simulink library "PUMATRC_lib"  (Simulink 6.0)
settings: Solver=ode45  SolverMode=SingleTasking  StartTime=0.0  StopTime=10.0  RelTol=1e-3
settings Model: LastModifiedBy=martin
settings OptimizationCC: BooleanDataType=off
settings DebuggingCC: SolverPrmCheckMsg=none
settings HardwareCC: TargetUnknown=on

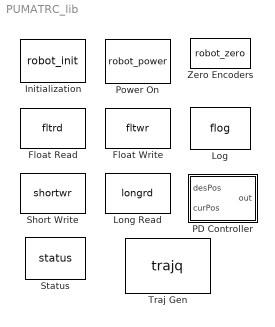
== system PUMATRC_lib ==
  Float Read : S-Function  Priority=10  FunctionName=fltrd  Parameters=option,channel,sampleTime  mask{option=TORQUE, channel=0, sampleTime=0}
      mask prompts: sampleTime "Sample Time"
      mask help: Reads a float value from OPTION offset and channel of Servo-To-Go board.
      mask StyleString: popup(TORQUE|TORQUE6|VOLTAGE|POSITION|POSITION6|STATUS|POT|POT6|INDEX|INDEX6|POWER|CALIB),edit,edit
      mask Display: port_label ('output',1,'val')
  Float Write : S-Function  Priority=10  FunctionName=fltwr  Parameters=option,channel,sampleTime  mask{option=TORQUE, channel=0, sampleTime=0}
      mask prompts: sampleTime "Sample Time"
      mask help: Writes a float value to OPTION offset and channel of Servo-To-Go board.
      mask StyleString: popup(TORQUE|TORQUE6|VOLTAGE|POSITION|POSITION6|STATUS|POT|POT6|INDEX|INDEX6|POWER|CALIB),edit,edit
      mask Display:
      | port_label('input',1,'val')
      | disp('')
  Initialization : S-Function  Priority=1  FunctionName=robot_init  Parameters=boardAddr  mask{boardAddr=0}
      mask prompts: boardAddr "Board Address(in decimal)"
      mask help: Initializes a Servo-To-Go board. Enter board address in decimal.
      mask Display: disp('Board\nInitialization')
  Log : S-Function  Priority=10  FunctionName=flog  Parameters=fileName,sampleTime  mask{fileName=0, sampleTime=0}
      mask prompts: fileName "Log Filename"; sampleTime "Sample Time"
      mask help: Values from the input are written to the filename at the specified period. The filename should be relative to the directory where model/code resides.
      mask Display:
      | port_label('input',1,'to File')
      | disp('')
  Long Read : S-Function  Priority=10  FunctionName=longrd  Parameters=option,channel,sampleTime  mask{option=TORQUE, channel=0, sampleTime=0}
      mask prompts: sampleTime "Sample Time"
      mask help: Writes a long value to OPTION offset and channel of Servo-To-Go board.
      mask StyleString: popup(TORQUE|TORQUE6|VOLTAGE|POSITION|POSITION6|STATUS|POT|POT6|INDEX|INDEX6|POWER|CALIB),edit,edit
      mask Display:
      | port_label('output',1,'val')
      | disp('')
  PD Controller : Subsystem  Priority=10  mask{Kp=0, Kd=0, T=0}
      mask prompts: T "Sample Time"
      mask help: Proportional-Derivative controller. Torque = Kp*(desPos- pos) - Kv*(time averaged velocity)
  Power On : S-Function  Priority=2  FunctionName=robot_power
      mask Display: disp('Power On')
  Short Write : S-Function  Priority=10  FunctionName=shortwr  Parameters=option,channel,sampleTime  mask{option=TORQUE, channel=0, sampleTime=0}
      mask prompts: sampleTime "Sample Time"
      mask help: Reads a short value from OPTION offset and channel of Servo-To-Go board.
      mask StyleString: popup(TORQUE|TORQUE6|VOLTAGE|POSITION|POSITION6|STATUS|POT|POT6|INDEX|INDEX6|POWER|CALIB),edit,edit
      mask Display:
      | port_label('input',1,'val')
      | disp('')
  Status : S-Function  FunctionName=status  Parameters=option,channel,sampleTime,  mask{option=TORQUE, channel=0, sampleTime=0}
      mask prompts: sampleTime "Sample Time"
      mask StyleString: popup(TORQUE|TORQUE6|VOLTAGE|POSITION|POSITION6|STATUS|POT|POT6|INDEX|INDEX6|POWER|CALIB|HAND|INDEX_BIT|ALL_INDEX_BITS|CLR_INDEX_BIT|CLR_INDEX_BITS|CLR_ADC_BIT ),edit,edit
      mask Display: port_label('output',1,'val')
  Traj Gen : S-Function  Priority=10  FunctionName=trajq  Parameters=sampleTime,jtMin,jtMax,calibFile,jtIncr  mask{sampleTime=0, jtMin=0, jtMax=0, calibFile=0, jtIncr=0}
      mask prompts: sampleTime "Sample Time"; jtMin "Joint Minimum Angles"; jtMax "Joint Maximum Angles"; calibFile "Calibration File Name"; jtIncr "Joint Increments"
      mask Display:
      | port_label('input',1,'theta')
      | port_label('input',2','enable')
      | port_label('output',1,'jt')
      | port_label('output',2,'stop')
  Zero Encoders : S-Function  Priority=3  FunctionName=robot_zero
      mask Display: disp('Zero\nEncoders')

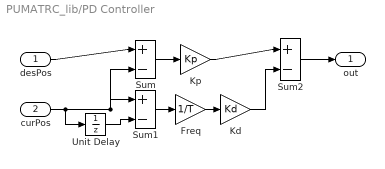
== system PUMATRC_lib/PD Controller ==
  desPos : Inport  Port=1  LatchInput=off
  curPos : Inport  Port=2  LatchInput=off
  Freq : Gain  Gain=1/T  SaturateOnIntegerOverflow=on
  Kd : Gain  Gain=Kd  SaturateOnIntegerOverflow=on
  Kp : Gain  Gain=Kp  SaturateOnIntegerOverflow=on
  Sum : Sum  Inputs=|+-  SaturateOnIntegerOverflow=on
  Sum1 : Sum  Inputs=|+-  SaturateOnIntegerOverflow=on
  Sum2 : Sum  Inputs=|+-  SaturateOnIntegerOverflow=on
  Unit Delay : UnitDelay  SampleTime=T
  out : Outport
  wires:
  Sum/1 -> Kp/1
  Unit Delay/1 -> Sum1/2
  Sum1/1 -> Freq/1
  Kp/1 -> Sum2/1
  Freq/1 -> Kd/1
  Kd/1 -> Sum2/2
  Sum2/1 -> out/1
  curPos/1 -> Sum1/1, Sum/2, Unit Delay/1
  desPos/1 -> Sum/1
